simulink model "process_with_signal"  (Simulink 7.6)
settings: Solver=ode45  StartTime=0.0  StopTime=50  RelTol=1e-3
settings Model: Creator=administrator  LastModifiedBy=administrator

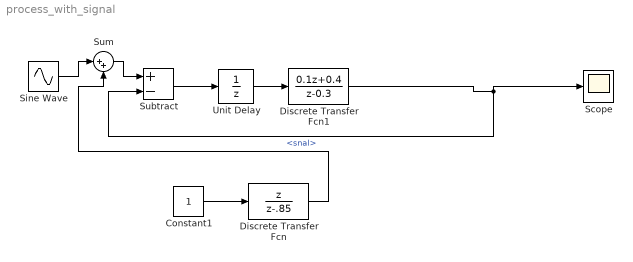
== system process_with_signal ==
  Constant1 : Constant
  Discrete Transfer Fcn : DiscreteTransferFcn  Numerator=[1 0]  Denominator=[1 -.85]
  Discrete Transfer Fcn1 : DiscreteTransferFcn  Numerator=[0.1 0.4]  Denominator=[1 -0.3]
  Scope : Scope
      settings: TimeRange=50
  Sine Wave : Sin  SampleTime=0
  Subtract : Sum  Inputs=+-
  Sum : Sum  Inputs=|++
  Unit Delay : UnitDelay  SampleTime=-1
  wires:
  Unit Delay/1 -> Discrete Transfer Fcn1/1
  Subtract/1 -> Unit Delay/1
  Discrete Transfer Fcn1/1 -> Subtract/2, Scope/1  "<snal>"
  Sine Wave/1 -> Sum/1
  Sum/1 -> Subtract/1
  Constant1/1 -> Discrete Transfer Fcn/1
  Discrete Transfer Fcn/1 -> Sum/2
